simulink model "VFT"  (Simulink 10.0)
settings: Solver=ode23tb  StartTime=0.0  StopTime=5  RelTol=1e-3  EnableMultiTasking=on
libraries: powerlib x12, powerlib_extras x6, simulink x1
settings Model: Creator=Asma  LastModifiedBy=bhisma
settings DataIOCC: LimitDataPoints=on  SignalLoggingSaveFormat=ModelDataLogs
settings OptimizationCC: ExpressionDepthLimit=2147483647
settings DebuggingCC: SolverPrmCheckMsg=warning  FcnCallInpInsideContextMsg=warning  StateNameClashWarn=warning
settings GRTTargetCC: GeneratePreprocessorConditionals=Disable all
settings ConfigComp: CovExternalEMLEnable=off
settings SimscapeCC: SimscapeNormalizeSystem=off

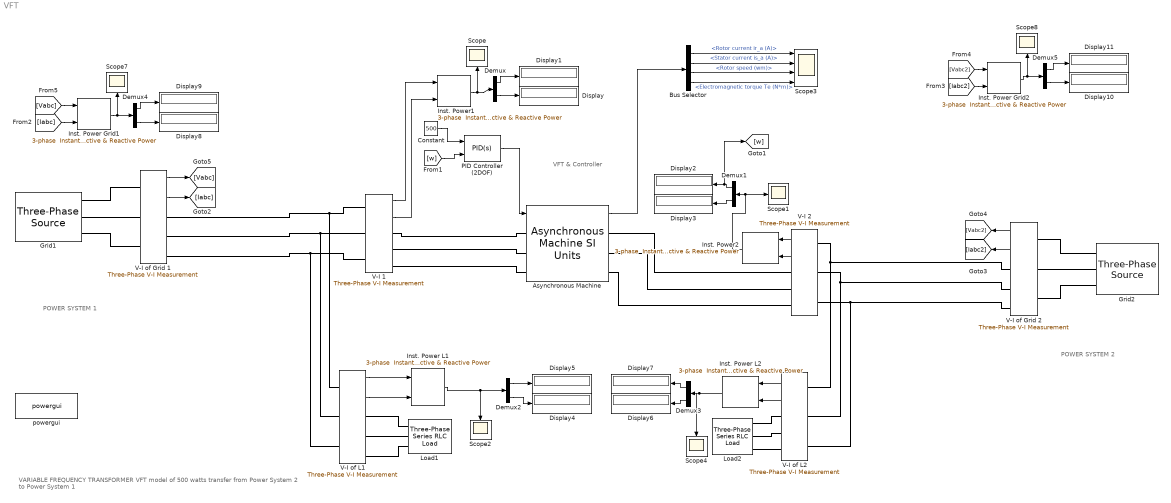
== system VFT ==
  note: POWER SYSTEM 1
  note: POWER SYSTEM 2
  note: VFT & Controller
  note: VARIABLE FREQUENCY TRANSFORMER
      | VFT model of 500 watts transfer from Power System 2
      | to Power System 1
  Asynchronous Machine : powerlib/Machines/Asynchronous Machine SI Units  SystemSampleTime=-1  PresetModel=No  MechanicalLoad=Speed w  ShowDetailedParameters=on  RotorType=Wound  ReferenceFrame=Rotor  NominalParameters=[3730 220 60 ]  Stator=[ 1.115 0.005974]  Rotor=[ 1.15 0.005974]  Lm=0.2037  Mechanical=[ 63.87 0 2]  PolePairs=2  InitialConditions=[1 0 0 0 0 0 0 0]  Units=SI  LoadFlowParameters=1492000  SimulateSaturation=off  Saturation=[14.03593122, 27.81365428, 53.79336849, 72.68890987, 97.98006896, 148.6815601, 215.7428561, 302.9841135, 428.7778367 ; 230, 322, 414, 460, 506, 552, 598, 644, 690]  TsPowergui=0  TsBlock=-1  IterativeModel=Forward Euler
      settings: SourceProductName=Simscape Electrical
  Bus Selector : BusSelector  OutputSignals=Rotor measurements.Rotor current ir_a (A),Stator measurements.Stator current is_a (A),Mechanical.Rotor speed (wm),Mechanical.Electromagnetic torque Te (N*m)
  Constant : Constant  Value=500
  Demux{,1..5} (6 alike) : Demux  Outputs=2
  Display{,1..11} (12 alike) : Display
  Grid1 : powerlib/Electrical Sources/Three-Phase Source  SystemSampleTime=-1  Voltage=220  PhaseAngle=0  Frequency=50  InternalConnection=Yg  SpecifyImpedance=off  Resistance=0.01  Inductance=0  ShortCircuitLevel=100e6  BaseVoltage=25e3  XRratio=7
      settings: SourceProductName=Simscape Electrical
  Grid2 : powerlib/Electrical Sources/Three-Phase Source  SystemSampleTime=-1  Voltage=220  PhaseAngle=0  Frequency=50  InternalConnection=Yg  SpecifyImpedance=off  Resistance=0.01  Inductance=0  ShortCircuitLevel=100e6  BaseVoltage=25e3  XRratio=7
      settings: SourceProductName=Simscape Electrical
  Inst. Power Grid1 : powerlib_extras/Measurements/3-phase  Instantaneous  Active & Reactive Power  SystemSampleTime=-1
      settings: SourceProductName=Simscape Electrical  SourceProductBaseCode=PS
  Inst. Power Grid2 : powerlib_extras/Measurements/3-phase  Instantaneous  Active & Reactive Power  SystemSampleTime=-1
      settings: SourceProductName=Simscape Electrical  SourceProductBaseCode=PS
  Inst. Power L1 : powerlib_extras/Measurements/3-phase  Instantaneous  Active & Reactive Power  SystemSampleTime=-1
      settings: SourceProductName=Simscape Electrical  SourceProductBaseCode=PS
  Inst. Power L2 : powerlib_extras/Measurements/3-phase  Instantaneous  Active & Reactive Power  SystemSampleTime=-1
      settings: SourceProductName=Simscape Electrical  SourceProductBaseCode=PS
  Inst. Power1 : powerlib_extras/Measurements/3-phase  Instantaneous  Active & Reactive Power  SystemSampleTime=-1
      settings: SourceProductName=Simscape Electrical  SourceProductBaseCode=PS
  Inst. Power2 : powerlib_extras/Measurements/3-phase  Instantaneous  Active & Reactive Power  SystemSampleTime=-1
      settings: SourceProductName=Simscape Electrical  SourceProductBaseCode=PS
  Load1 : powerlib/Elements/Three-Phase Series RLC Load  PhysicalDomain=powersysdomain  SubClassName=unknown  LeftPortType=p1  RightPortType=p1  LConnTagsString=A|B|C  Configuration=Y (grounded)  NominalVoltage=220  NominalFrequency=50  ActivePower=1000  InductivePower=0  CapacitivePower=0  Measurements=None
      settings: SourceProductName=Simscape Electrical
  Load2 : powerlib/Elements/Three-Phase Series RLC Load  PhysicalDomain=powersysdomain  SubClassName=unknown  LeftPortType=p1  RightPortType=p1  LConnTagsString=A|B|C  Configuration=Y (grounded)  NominalVoltage=220  NominalFrequency=50  ActivePower=4000  InductivePower=0  CapacitivePower=0  Measurements=None
      settings: SourceProductName=Simscape Electrical
  PID Controller (2DOF) : simulink/Continuous/PID Controller (2DOF)  SystemSampleTime=-1  Controller=PID  TimeDomain=Continuous-time  SampleTime=1  IntegratorMethod=Forward Euler  FilterMethod=Forward Euler  Form=Parallel  P=.1  I=.01  D=0  N=100  b=1  c=1  InitialConditionSource=internal  InitialConditionForIntegrator=0  InitialConditionForFilter=0  ExternalReset=none  LimitOutput=off  UpperSaturationLimit=inf  LowerSaturationLimit=-inf  LinearizeAsGain=on  AntiWindupMode=none  Kb=1  TrackingMode=off  Kt=1  PParamMin=[]  PParamMax=[]  IParamMin=[]  IParamMax=[]  DParamMin=[]  DParamMax=[]  NParamMin=[]  NParamMax=[]  bParamMin=[]  bParamMax=[]  cParamMin=[]  cParamMax=[]  KbParamMin=[]  KbParamMax=[]  KtParamMin=[]  KtParamMax=[]  POutMin=[]  POutMax=[]  IOutMin=[]  IOutMax=[]  DOutMin=[]  DOutMax=[]  NOutMin=[]  NOutMax=[]  bOutMin=[]  bOutMax=[]  cOutMin=[]  cOutMax=[]  KbOutMin=[]  KbOutMax=[]  KtOutMin=[]  KtOutMax=[]  IntegratorOutMin=[]  IntegratorOutMax=[]  FilterOutMin=[]  FilterOutMax=[]  SumOutMin=[]  SumOutMax=[]  Sum1OutMin=[]  Sum1OutMax=[]  Sum2OutMin=[]  Sum2OutMax=[]  Sum3OutMin=[]  Sum3OutMax=[]  SumI1OutMin=[]  SumI1OutMax=[]  SumI2OutMin=[]  SumI2OutMax=[]  SumI3OutMin=[]  SumI3OutMax=[]  SumDOutMin=[]  SumDOutMax=[]  SaturationOutMin=[]  SaturationOutMax=[]  IntegratorContinuousStateAttributes=''  IntegratorStateMustResolveToSignalObject=off  IntegratorRTWStateStorageClass=Auto  FilterContinuousStateAttributes=''  FilterStateMustResolveToSignalObject=off  FilterRTWStateStorageClass=Auto
  Scope{,1..2,4,7..8} (6 alike) : Scope
  Scope3 : Scope  NumInputPorts=4
  V-I 1 : powerlib/Measurements/Three-Phase V-I Measurement  SystemSampleTime=-1  VoltageMeasurement=phase-to-ground  SetLabelV=off  LabelV=Vabc  Vpu=off  VpuLL=off  CurrentMeasurement=yes  SetLabelI=off  LabelI=Iabc  Ipu=off  Pbase=100e6  Vbase=500e3  OutputType=Complex  PhasorSimulation=off  PSBequivalent=0
      link override Model/VI/Ia: GotoTag=LibraryTag_Ia
      link override Model/VI/Ib: GotoTag=LibraryTag_Ib
      link override Model/VI/Ic: GotoTag=LibraryTag_Ic
      link override Model/VI/Va: GotoTag=LibraryTag_Va
      link override Model/VI/Vb: GotoTag=LibraryTag_Vb
      link override Model/VI/Vc: GotoTag=LibraryTag_Vc
      settings: SourceProductName=Simscape Electrical
  V-I 2 : powerlib/Measurements/Three-Phase V-I Measurement  SystemSampleTime=-1  VoltageMeasurement=phase-to-ground  SetLabelV=off  LabelV=Vabc  Vpu=off  VpuLL=off  CurrentMeasurement=yes  SetLabelI=off  LabelI=Iabc  Ipu=off  Pbase=100e6  Vbase=500e3  OutputType=Complex  PhasorSimulation=off  PSBequivalent=0
      link override Model/VI/Ia: GotoTag=LibraryTag_Ia
      link override Model/VI/Ib: GotoTag=LibraryTag_Ib
      link override Model/VI/Ic: GotoTag=LibraryTag_Ic
      link override Model/VI/Va: GotoTag=LibraryTag_Va
      link override Model/VI/Vb: GotoTag=LibraryTag_Vb
      link override Model/VI/Vc: GotoTag=LibraryTag_Vc
      settings: SourceProductName=Simscape Electrical
  V-I of Grid 1 : powerlib/Measurements/Three-Phase V-I Measurement  SystemSampleTime=-1  VoltageMeasurement=phase-to-ground  SetLabelV=off  LabelV=Vabc  Vpu=off  VpuLL=off  CurrentMeasurement=yes  SetLabelI=off  LabelI=Iabc  Ipu=off  Pbase=100e6  Vbase=500e3  OutputType=Complex  PhasorSimulation=off  PSBequivalent=0
      link override Model/VI/Ia: GotoTag=LibraryTag_Ia
      link override Model/VI/Ib: GotoTag=LibraryTag_Ib
      link override Model/VI/Ic: GotoTag=LibraryTag_Ic
      link override Model/VI/Va: GotoTag=LibraryTag_Va
      link override Model/VI/Vb: GotoTag=LibraryTag_Vb
      link override Model/VI/Vc: GotoTag=LibraryTag_Vc
      settings: SourceProductName=Simscape Electrical
  V-I of Grid 2 : powerlib/Measurements/Three-Phase V-I Measurement  SystemSampleTime=-1  VoltageMeasurement=phase-to-ground  SetLabelV=off  LabelV=Vabc  Vpu=off  VpuLL=off  CurrentMeasurement=yes  SetLabelI=off  LabelI=Iabc  Ipu=off  Pbase=100e6  Vbase=500e3  OutputType=Complex  PhasorSimulation=off  PSBequivalent=0
      link override Model/VI/Ia: GotoTag=LibraryTag_Ia
      link override Model/VI/Ib: GotoTag=LibraryTag_Ib
      link override Model/VI/Ic: GotoTag=LibraryTag_Ic
      link override Model/VI/Va: GotoTag=LibraryTag_Va
      link override Model/VI/Vb: GotoTag=LibraryTag_Vb
      link override Model/VI/Vc: GotoTag=LibraryTag_Vc
      settings: SourceProductName=Simscape Electrical
  "V-I of L1 " : powerlib/Measurements/Three-Phase V-I Measurement  SystemSampleTime=-1  VoltageMeasurement=phase-to-ground  SetLabelV=off  LabelV=Vabc  Vpu=off  VpuLL=off  CurrentMeasurement=yes  SetLabelI=off  LabelI=Iabc  Ipu=off  Pbase=100e6  Vbase=500e3  OutputType=Complex  PhasorSimulation=off  PSBequivalent=0
      link override Model/VI/Ia: GotoTag=LibraryTag_Ia
      link override Model/VI/Ib: GotoTag=LibraryTag_Ib
      link override Model/VI/Ic: GotoTag=LibraryTag_Ic
      link override Model/VI/Va: GotoTag=LibraryTag_Va
      link override Model/VI/Vb: GotoTag=LibraryTag_Vb
      link override Model/VI/Vc: GotoTag=LibraryTag_Vc
      settings: SourceProductName=Simscape Electrical
  V-I of L2 : powerlib/Measurements/Three-Phase V-I Measurement  SystemSampleTime=-1  VoltageMeasurement=phase-to-ground  SetLabelV=off  LabelV=Vabc  Vpu=off  VpuLL=off  CurrentMeasurement=yes  SetLabelI=off  LabelI=Iabc  Ipu=off  Pbase=100e6  Vbase=500e3  OutputType=Complex  PhasorSimulation=off  PSBequivalent=0
      link override Model/VI/Ia: GotoTag=LibraryTag_Ia
      link override Model/VI/Ib: GotoTag=LibraryTag_Ib
      link override Model/VI/Ic: GotoTag=LibraryTag_Ic
      link override Model/VI/Va: GotoTag=LibraryTag_Va
      link override Model/VI/Vb: GotoTag=LibraryTag_Vb
      link override Model/VI/Vc: GotoTag=LibraryTag_Vc
      settings: SourceProductName=Simscape Electrical
  powergui : powerlib/powergui  Priority=1  SystemSampleTime=-1  SimulationMode=Continuous  SampleTime=50e-5  frequency=60  SPID=off  DisableSnubberDevices=off  DisableRonSwitches=off  DisableVfSwitches=off  SwTol=0  Interpol=off  frequencyindice=60  echomessages=off  HookPort=off  DisplayEquations=off  FunctionMessages=off  EnableUseOfTLC=off  x0status=blocks  RestoreLinks=warning  ResistiveCurrentMeasurement=off  Frange=[0:2:500]  Ylog=off  Xlog=on  ShowGrid=off  save=off  variable=ZData  structure=ScopeData8  ZoomFFT=off  StartTime=2.5  cycles=1  DisplayStyle=2  fundamental=50  FreqAxis=off  MaxFrequency=1000  frequencyindicesteady=1  RmsSteady=1  display=off  Ts=0  methode=off
      settings: SourceProductName=Simscape Electrical
  wires:
  [Vabc] -> Inst. Power Grid1/1
  V-I of Grid 1/1 -> [Vabc]
  V-I of Grid 1/2 -> [Iabc]
  Inst. Power2/1 -> Demux1/1, Scope1/1
  Demux1/2 -> Display3/1
  Demux1/1 -> [w], Display2/1
  V-I 2/2 -> Inst. Power2/2
  V-I 2/1 -> Inst. Power2/1
  [Vabc2] -> Inst. Power Grid2/1
  V-I of Grid 2/1 -> [Vabc2]
  V-I of Grid 2/2 -> [Iabc2]
  Inst. Power L2/1 -> Demux3/1, Scope4/1
  V-I of L2/2 -> Inst. Power L2/2
  V-I of L2/1 -> Inst. Power L2/1
  [Iabc2] -> Inst. Power Grid2/2
  [Iabc] -> Inst. Power Grid1/2
  Demux5/2 -> Display10/1
  Demux5/1 -> Display11/1
  Inst. Power Grid2/1 -> Demux5/1, Scope8/1
  Demux4/2 -> Display8/1
  Demux4/1 -> Display9/1
  Inst. Power Grid1/1 -> Demux4/1, Scope7/1
  "V-I of L1 "/1 -> Inst. Power L1/1
  Inst. Power L1/1 -> Demux2/1, Scope2/1
  "V-I of L1 "/2 -> Inst. Power L1/2
  Demux3/2 -> Display6/1
  Demux3/1 -> Display7/1
  Demux2/2 -> Display4/1
  Demux2/1 -> Display5/1
  Bus Selector/4 -> Scope3/4  "<Electromagnetic torque Te (N*m)>"
  Bus Selector/3 -> Scope3/3  "<Rotor speed (wm)>"
  Bus Selector/2 -> Scope3/2  "<Stator current is_a (A)>"
  Bus Selector/1 -> Scope3/1  "<Rotor current ir_a (A)>"
  Asynchronous Machine/1 -> Bus Selector/1
  Demux/2 -> Display/1
  Demux/1 -> Display1/1
  Inst. Power1/1 -> Demux/1, Scope/1
  V-I 1/2 -> Inst. Power1/2
  V-I 1/1 -> Inst. Power1/1
  Constant/1 -> PID Controller (2DOF)/1
  [w] -> PID Controller (2DOF)/2
  PID Controller (2DOF)/1 -> Asynchronous Machine/1
  connections:
  Grid1/RConn3 -- V-I of Grid 1/LConn3
  Grid1/RConn2 -- V-I of Grid 1/LConn2
  Grid1/RConn1 -- V-I of Grid 1/LConn1
  V-I of Grid 2/LConn3 -- Grid2/RConn3
  V-I of Grid 2/LConn2 -- Grid2/RConn2
  V-I of Grid 2/LConn1 -- Grid2/RConn1
  Load2/LConn3 -- V-I of L2/RConn3
  Load2/LConn2 -- V-I of L2/RConn2
  Load2/LConn1 -- V-I of L2/RConn1
  Asynchronous Machine/RConn3 -- V-I 2/RConn3
  Asynchronous Machine/RConn2 -- V-I 2/RConn2
  Asynchronous Machine/RConn1 -- V-I 2/RConn1
  V-I 1/RConn3 -- Asynchronous Machine/LConn3
  V-I 1/RConn2 -- Asynchronous Machine/LConn2
  V-I 1/RConn1 -- Asynchronous Machine/LConn1
  "V-I of L1 "/RConn3 -- Load1/LConn3
  "V-I of L1 "/RConn1 -- Load1/LConn1
  "V-I of L1 "/RConn2 -- Load1/LConn2
  V-I of Grid 2/RConn3 -- V-I 2/LConn3 -- V-I of L2/LConn3
  V-I of Grid 2/RConn2 -- V-I 2/LConn2 -- V-I of L2/LConn2
  V-I of Grid 2/RConn1 -- V-I 2/LConn1 -- V-I of L2/LConn1
  V-I of Grid 1/RConn3 -- V-I 1/LConn3 -- "V-I of L1 "/LConn3
  V-I of Grid 1/RConn2 -- V-I 1/LConn2 -- "V-I of L1 "/LConn2
  V-I of Grid 1/RConn1 -- V-I 1/LConn1 -- "V-I of L1 "/LConn1
